simulink library "thermochemical"  (R2017b)
settings: Solver=VariableStepAuto  StartTime=0.0  StopTime=10.0  RelTol=1e-3
values from neighbouring files (symbols this model uses):
  c = conversion_factors()    [blk_clausius_clapeyron.m]    (also in blk_clausius_clapeyron_no_popup.m; blk_cold_room_closed_dry_air.m; blk_reactor_BaCl2_NH3_no_walls.m; blk_reactor_BaCl2_NH3_no_walls_state_space.m)
  cp = metal.cp    [blk_wall_simple.m]    (also in get_metal_properties.m = 390)
  fluid = get_param(blk,'fluid')    [blk_thermodynamic_properties_nonsaturated.m]    (also in blk_thermodynamic_properties_nonsaturated_interpreted.m; blk_thermodynamic_properties_saturated.m; blk_thermodynamic_properties_saturated_interpreted.m; blk_thermodynamic_properties_saturated_mix.m)
  gas = get_material_properties(x.gasName)    [blk_reactor_BaCl2_NH3_cylindrical_no_walls_fun1.m]
  h = get_param(gcb,'ObjectParameters')    [get_param_eval.m]
  rho = metal.rho    [blk_wall_simple.m]    (also in get_metal_properties.m = 8940)
  s = solve(eq,dx,'ReturnConditions',true)    [LMTD_inv.m]    (also in blk_wall_simple.m = get_param_eval(blk,'s'))
  u_gas_at_T_ref = -R * T_ref    [blk_reactor_BaCl2_NH3_no_walls.m]    (also in blk_reactor_BaCl2_NH3_no_walls_state_space.m)
undefined symbols (not defined in the file or in its folder): b_motor, BaCl2, beta, CoolProp, cP_binder, cP_gas, cP_s0, cv, dh_r_0, ENG, heat_exchanger_epsilonNTU_inv_simulink, heat_exchanger_epsilonNTU_simulink, J_motor, K_cin, kappa, Km_motor, La_motor, lookup2D_BreakPoint2, M_binder, N_binder, N_gas_free_volume_init, N_salt, NH3, nh3_v3, nu, P, phase, PID_D_motor, PID_I_motor, PID_P_motor, Ra_motor, Reactor_phase, T, T1, T2, T_init, Tr_init, Tr_ref, U_binder_at_Tr_ref, U_salt_at_X0_Tr_ref, Ur_init, V_void, Valve_regime, Vmax_motor, w_init_motor, X_init
libraries: thermochemical x247, simulink x54, dspsigops x3
(part 11 of 12)

== system thermochemical/Reactors/Reactor, BaCl2//NH3, state-space form, [Tr, Ng, X] as state variables, no algebraic loops, ideal gas in void volume, ideal gas in salt/Reactor, BaCl2//NH3, no walls, state-space form, [Tr, Ng, X] as state variables, no algebraic loops, ideal gas in void volume/Reactor, no walls, state space form/Reactor state-space functions/f3/f3 ==
  In6 : Inport
  In1 : Inport  Port=2
  In2 : Inport  Port=3
  Gain4 : Gain  Gain=nu*N_salt
  Gain7 : Gain  Gain=1/V_void
  Ideal gas equation of state : thermochemical/Thermodynamic fluid properties/Ideal gas equation of state  sel=P(T,rho)  R=8.3145  Pa_to_bar=1e-5  bar_to_Pa=1e5
      settings: SourceProductName=@ Thermochemical
  "Reaction kinetic, differential equation" : Subsystem
  Sum2 : Sum  Inputs=|+-
  Out2 : Outport
  wires:
  "Reaction kinetic, differential equation"/1(Out2) -> Out2/1  "dX/dt (1/sec)"
  Ideal gas equation of state/1 -> "Reaction kinetic, differential equation"/2(In2)
  Sum2/1 -> Gain7/1  "Ngas,void"
  Gain7/1 -> Ideal gas equation of state/2
  Gain4/1 -> Sum2/2
  In6/1 -> "Reaction kinetic, differential equation"/1(In1), Ideal gas equation of state/1  "T (K)"
  In1/1 -> Sum2/1  "Ngas,total (mol)"
  In2/1 -> Gain4/1, "Reaction kinetic, differential equation"/3(In3)  "X (0..1)"

== system thermochemical/Reactors/Reactor, BaCl2//NH3, state-space form, [Tr, Ng, X] as state variables, no algebraic loops, real gas in void volume, ideal gas in salt/Reactor, BaCl2//NH3, no walls, state-space form, [Tr, Ng, X] as state variables, no algebraic loops, real gas in void volume, ideal gas in salt/Reactor, no walls, state space form/Reactor state-space functions/f1/denominator ==
  In6 : Inport
  In3 : Inport  Port=2
  In4 : Inport  Port=3
  Gain4 : Gain  Gain=nu*N_salt
  Gain7 : Gain  Gain=1/V_void
  K1 : Constant  Value=N_salt*cP_s0 + N_binder*M_binder*cP_binder  VectorParams1D=off
  K2 : Constant  Value=cP_gas  VectorParams1D=off
  Product1 : Product
  Product4 : Product
  Sum : Sum  Inputs=3
  Sum5 : Sum  Inputs=|+-
  Thermodynamic property (non-saturated)1 : thermochemical/Thermodynamic fluid properties/Thermodynamic  property (non-saturated)  sel=cv(T,rho)  fluid=fluid  reciprocVar=-1  lookup2D_BreakPoint1=fluid.no_sat.T_rho_indep.var_indep.T  lookup2D_BreakPoint2=fluid.no_sat.T_rho_indep.var_indep.rho_molar  lookup2D_Data=fluid.no_sat.T_rho_indep.var_dep.Cv_molar
      settings: SourceProductName=@ Thermochemical
  Thermodynamic property (non-saturated)2 : thermochemical/Thermodynamic fluid properties/Thermodynamic  property (non-saturated)  sel=cp(T,rho)  fluid=fluid  reciprocVar=-1  lookup2D_BreakPoint1=fluid.no_sat.T_rho_indep.var_indep.T  lookup2D_BreakPoint2=fluid.no_sat.T_rho_indep.var_indep.rho_molar  lookup2D_Data=fluid.no_sat.T_rho_indep.var_dep.Cp_molar
      settings: SourceProductName=@ Thermochemical
  Out2 : Outport
  wires:
  K1/1 -> Sum/1  "(J/K)"
  Sum/1 -> Out2/1  "denominator (J/K)"
  Sum5/1 -> Gain7/1, Product4/2  "Ngas,void"
  In4/1 -> Gain4/1  "X (0..1)"
  In3/1 -> Sum5/1  "Ngas,total (mol)"
  Gain7/1 -> Thermodynamic property (non-saturated)2/2, Thermodynamic property (non-saturated)1/2  "rho (mol/m3)"
  In6/1 -> Thermodynamic property (non-saturated)2/1, Thermodynamic property (non-saturated)1/1  "T (K)"
  Thermodynamic property (non-saturated)1/1 -> Product4/1
  Product4/1 -> Sum/2  "(J/K)"
  Gain4/1 -> Product1/1, Sum5/2  "(mol gas/mol salt * mol salt = mol gas)"
  Thermodynamic property (non-saturated)2/1 -> ?
  Product1/1 -> Sum/3  "(J/K)"
  K2/1 -> Product1/2

== system thermochemical/Reactors/Reactor, BaCl2//NH3, state-space form, [Tr, Ng, X] as state variables, no algebraic loops, real gas in void volume, ideal gas in salt/Reactor, BaCl2//NH3, no walls, state-space form, [Tr, Ng, X] as state variables, no algebraic loops, real gas in void volume, ideal gas in salt/Reactor, no walls, state space form/Reactor state-space functions/f1/f1 ==
  In6 : Inport
  In1 : Inport  Port=2
  In2 : Inport  Port=3
  Gain4 : Gain  Gain=nu*N_salt
  Gain7 : Gain  Gain=1/V_void
  Sum2 : Sum  Inputs=|+-
  Thermodynamic property (non-saturated)1 : thermochemical/Thermodynamic fluid properties/Thermodynamic  property (non-saturated)  sel=h(T,rho)  fluid=fluid  reciprocVar=-1  lookup2D_BreakPoint1=fluid.no_sat.T_rho_indep.var_indep.T  lookup2D_BreakPoint2=fluid.no_sat.T_rho_indep.var_indep.rho_molar  lookup2D_Data=fluid.no_sat.T_rho_indep.var_dep.h_molar
      settings: SourceProductName=@ Thermochemical
  Out2 : Outport
  wires:
  Thermodynamic property (non-saturated)1/1 -> Out2/1  "h gas (J/mol)"
  Sum2/1 -> Gain7/1  "Ngas,void"
  Gain7/1 -> Thermodynamic property (non-saturated)1/2
  Gain4/1 -> Sum2/2
  In6/1 -> Thermodynamic property (non-saturated)1/1  "T (K)"
  In1/1 -> Sum2/1  "Ngas,total (mol)"
  In2/1 -> Gain4/1  "X (0..1)"

== system thermochemical/Reactors/Reactor, BaCl2//NH3, state-space form, [Tr, Ng, X] as state variables, no algebraic loops, real gas in void volume, ideal gas in salt/Reactor, BaCl2//NH3, no walls, state-space form, [Tr, Ng, X] as state variables, no algebraic loops, real gas in void volume, ideal gas in salt/Reactor, no walls, state space form/Reactor state-space functions/f1/f2 ==
  In6 : Inport
  In1 : Inport  Port=2
  In2 : Inport  Port=3
  Gain4 : Gain  Gain=nu*N_salt
  Gain7 : Gain  Gain=1/V_void
  Math Function : Math  Operator=reciprocal  SaturateOnIntegerOverflow=on
  Pressure conversion : thermochemical/Conversions/Pressure conversion  sel=bar --> Pa
      settings: SourceProductName=@ Thermochemical
  Product1 : Product
  Product4 : Product  Inputs=**/
  Sum5 : Sum  Inputs=|+-
  Sum6 : Sum  Inputs=|+-
  Sum7 : Sum  Inputs=|+-
  Thermodynamic property (non-saturated) : thermochemical/Thermodynamic fluid properties/Thermodynamic  property (non-saturated)  sel=u(T,rho)  fluid=fluid  reciprocVar=-1  lookup2D_BreakPoint1=fluid.no_sat.T_rho_indep.var_indep.T  lookup2D_BreakPoint2=fluid.no_sat.T_rho_indep.var_indep.rho_molar  lookup2D_Data=fluid.no_sat.T_rho_indep.var_dep.u_molar
      settings: SourceProductName=@ Thermochemical
  Thermodynamic property (non-saturated)1 : thermochemical/Thermodynamic fluid properties/Thermodynamic  property (non-saturated)  sel=beta(T,rho)  fluid=fluid  reciprocVar=-1  lookup2D_BreakPoint1=fluid.no_sat.T_rho_indep.var_indep.T  lookup2D_BreakPoint2=fluid.no_sat.T_rho_indep.var_indep.rho_molar  lookup2D_Data=fluid.no_sat.T_rho_indep.var_dep.beta
      settings: SourceProductName=@ Thermochemical
  Thermodynamic property (non-saturated)2 : thermochemical/Thermodynamic fluid properties/Thermodynamic  property (non-saturated)  sel=kappa(T,rho)  fluid=fluid  reciprocVar=-1  lookup2D_BreakPoint1=fluid.no_sat.T_rho_indep.var_indep.T  lookup2D_BreakPoint2=fluid.no_sat.T_rho_indep.var_indep.rho_molar  lookup2D_Data=fluid.no_sat.T_rho_indep.var_dep.kappa
      settings: SourceProductName=@ Thermochemical
  Thermodynamic property (non-saturated)3 : thermochemical/Thermodynamic fluid properties/Thermodynamic  property (non-saturated)  sel=P(T,rho)  fluid=fluid  reciprocVar=-1  lookup2D_BreakPoint1=fluid.no_sat.T_rho_indep.var_indep.T  lookup2D_BreakPoint2=fluid.no_sat.T_rho_indep.var_indep.rho_molar  lookup2D_Data=fluid.no_sat.T_rho_indep.var_dep.P
      settings: SourceProductName=@ Thermochemical
  Out2 : Outport
  wires:
  Pressure conversion/1 -> Sum7/2
  In6/1 -> Product4/1, Thermodynamic property (non-saturated)3/1, Thermodynamic property (non-saturated)2/1, Thermodynamic property (non-saturated)1/1, Thermodynamic property (non-saturated)/1  "T (K)"
  In1/1 -> Sum5/1  "Ngas,total (mol)"
  Gain4/1 -> Sum5/2
  In2/1 -> Gain4/1  "X (0..1)"
  Sum5/1 -> Gain7/1  "Ngas,void"
  Gain7/1 -> Math Function/1, Thermodynamic property (non-saturated)2/2, Thermodynamic property (non-saturated)3/2, Thermodynamic property (non-saturated)1/2, Thermodynamic property (non-saturated)/2  "rho (mol/m3)"
  Thermodynamic property (non-saturated)/1 -> Sum6/1  "u gas (J/mol)"
  Thermodynamic property (non-saturated)1/1 -> Product4/2
  Thermodynamic property (non-saturated)2/1 -> Product4/3
  Product4/1 -> Sum7/1
  Thermodynamic property (non-saturated)3/1 -> Pressure conversion/1
  Math Function/1 -> Product1/1
  Sum7/1 -> Product1/2
  Product1/1 -> Sum6/2  "(J/mol)"
  Sum6/1 -> Out2/1  "u - 1/rho*(T*beta/kappa-P) (J/mol)"

== system thermochemical/Reactors/Reactor, BaCl2//NH3, state-space form, [Tr, Ng, X] as state variables, no algebraic loops, real gas in void volume, ideal gas in salt/Reactor, BaCl2//NH3, no walls, state-space form, [Tr, Ng, X] as state variables, no algebraic loops, real gas in void volume, ideal gas in salt/Reactor, no walls, state space form/Reactor state-space functions/f1/f3 ==
  In6 : Inport
  In1 : Inport  Port=2
  In2 : Inport  Port=3
  Gain4 : Gain  Gain=nu*N_salt
  Gain7 : Gain  Gain=1/V_void
  "Reaction kinetic, differential equation" : Subsystem
  Sum2 : Sum  Inputs=|+-
  Thermodynamic property (non-saturated)1 : thermochemical/Thermodynamic fluid properties/Thermodynamic  property (non-saturated)  sel=P(T,rho)  fluid=fluid  reciprocVar=-1  lookup2D_BreakPoint1=fluid.no_sat.T_rho_indep.var_indep.T  lookup2D_BreakPoint2=fluid.no_sat.T_rho_indep.var_indep.rho_molar  lookup2D_Data=fluid.no_sat.T_rho_indep.var_dep.P
      settings: SourceProductName=@ Thermochemical
  Out2 : Outport
  wires:
  In2/1 -> "Reaction kinetic, differential equation"/3(In3), Gain4/1  "X (0..1)"
  In1/1 -> Sum2/1  "Ngas,total (mol)"
  In6/1 -> "Reaction kinetic, differential equation"/1(In1), Thermodynamic property (non-saturated)1/1  "T (K)"
  Gain4/1 -> Sum2/2
  Gain7/1 -> Thermodynamic property (non-saturated)1/2
  Sum2/1 -> Gain7/1  "Ngas,void"
  Thermodynamic property (non-saturated)1/1 -> "Reaction kinetic, differential equation"/2(In2)
  "Reaction kinetic, differential equation"/1(Out2) -> Out2/1  "dX/dt (1/sec)"

== system thermochemical/Reactors/Reactor, BaCl2//NH3, state-space form, [Tr, Ng, X] as state variables, no algebraic loops, real gas in void volume, real gas in salt/Reactor, BaCl2//NH3, no walls, state-space form, [Tr, Ng, X] as state variables, no algebraic loops, real gas in void volume, real gas in salt/Reactor, no walls, state space form/Reactor state-space functions/f1/denominator ==
  In6 : Inport
  In3 : Inport  Port=2
  In4 : Inport  Port=3
  Gain4 : Gain  Gain=nu*N_salt
  Gain7 : Gain  Gain=1/V_void
  K1 : Constant  Value=N_salt*cP_s0 + N_binder*M_binder*cP_binder  VectorParams1D=off
  Product1 : Product
  Product4 : Product
  Sum : Sum  Inputs=3
  Sum5 : Sum  Inputs=|+-
  Thermodynamic property (non-saturated)1 : thermochemical/Thermodynamic fluid properties/Thermodynamic  property (non-saturated)  sel=cv(T,rho)  fluid=fluid  reciprocVar=-1  lookup2D_BreakPoint1=fluid.no_sat.T_rho_indep.var_indep.T  lookup2D_BreakPoint2=fluid.no_sat.T_rho_indep.var_indep.rho_molar  lookup2D_Data=fluid.no_sat.T_rho_indep.var_dep.Cv_molar
      settings: SourceProductName=@ Thermochemical
  Thermodynamic property (non-saturated)2 : thermochemical/Thermodynamic fluid properties/Thermodynamic  property (non-saturated)  sel=cp(T,rho)  fluid=fluid  reciprocVar=-1  lookup2D_BreakPoint1=fluid.no_sat.T_rho_indep.var_indep.T  lookup2D_BreakPoint2=fluid.no_sat.T_rho_indep.var_indep.rho_molar  lookup2D_Data=fluid.no_sat.T_rho_indep.var_dep.Cp_molar
      settings: SourceProductName=@ Thermochemical
  Out2 : Outport
  wires:
  Product1/1 -> Sum/3  "(J/K)"
  Thermodynamic property (non-saturated)2/1 -> Product1/2
  Gain4/1 -> Sum5/2, Product1/1  "(mol gas/mol salt * mol salt = mol gas)"
  Product4/1 -> Sum/2  "(J/K)"
  Thermodynamic property (non-saturated)1/1 -> Product4/1
  In6/1 -> Thermodynamic property (non-saturated)1/1, Thermodynamic property (non-saturated)2/1  "T (K)"
  Gain7/1 -> Thermodynamic property (non-saturated)1/2, Thermodynamic property (non-saturated)2/2  "rho (mol/m3)"
  In3/1 -> Sum5/1  "Ngas,total (mol)"
  In4/1 -> Gain4/1  "X (0..1)"
  Sum5/1 -> Product4/2, Gain7/1  "Ngas,void"
  Sum/1 -> Out2/1  "denominator (J/K)"
  K1/1 -> Sum/1  "(J/K)"

== system thermochemical/Reactors/Reactor, BaCl2//NH3, state-space form, [Tr, Ng, X] as state variables, no algebraic loops, real gas in void volume, real gas in salt/Reactor, BaCl2//NH3, no walls, state-space form, [Tr, Ng, X] as state variables, no algebraic loops, real gas in void volume, real gas in salt/Reactor, no walls, state space form/Reactor state-space functions/f1/f1 ==
  In6 : Inport
  In1 : Inport  Port=2
  In2 : Inport  Port=3
  Gain4 : Gain  Gain=nu*N_salt
  Gain7 : Gain  Gain=1/V_void
  Sum2 : Sum  Inputs=|+-
  Thermodynamic property (non-saturated)1 : thermochemical/Thermodynamic fluid properties/Thermodynamic  property (non-saturated)  sel=h(T,rho)  fluid=fluid  reciprocVar=-1  lookup2D_BreakPoint1=fluid.no_sat.T_rho_indep.var_indep.T  lookup2D_BreakPoint2=fluid.no_sat.T_rho_indep.var_indep.rho_molar  lookup2D_Data=fluid.no_sat.T_rho_indep.var_dep.h_molar
      settings: SourceProductName=@ Thermochemical
  Out2 : Outport
  wires:
  In2/1 -> Gain4/1  "X (0..1)"
  In1/1 -> Sum2/1  "Ngas,total (mol)"
  In6/1 -> Thermodynamic property (non-saturated)1/1  "T (K)"
  Gain4/1 -> Sum2/2
  Gain7/1 -> Thermodynamic property (non-saturated)1/2
  Sum2/1 -> Gain7/1  "Ngas,void"
  Thermodynamic property (non-saturated)1/1 -> Out2/1  "h gas (J/mol)"

== system thermochemical/Reactors/Reactor, BaCl2//NH3, state-space form, [Tr, Ng, X] as state variables, no algebraic loops, real gas in void volume, real gas in salt/Reactor, BaCl2//NH3, no walls, state-space form, [Tr, Ng, X] as state variables, no algebraic loops, real gas in void volume, real gas in salt/Reactor, no walls, state space form/Reactor state-space functions/f1/f2 ==
  In6 : Inport
  In1 : Inport  Port=2
  In2 : Inport  Port=3
  Gain4 : Gain  Gain=nu*N_salt
  Gain7 : Gain  Gain=1/V_void
  Math Function : Math  Operator=reciprocal  SaturateOnIntegerOverflow=on
  Pressure conversion : thermochemical/Conversions/Pressure conversion  sel=bar --> Pa
      settings: SourceProductName=@ Thermochemical
  Product1 : Product
  Product4 : Product  Inputs=**/
  Sum5 : Sum  Inputs=|+-
  Sum6 : Sum  Inputs=|+-
  Sum7 : Sum  Inputs=|+-
  Thermodynamic property (non-saturated) : thermochemical/Thermodynamic fluid properties/Thermodynamic  property (non-saturated)  sel=u(T,rho)  fluid=fluid  reciprocVar=-1  lookup2D_BreakPoint1=fluid.no_sat.T_rho_indep.var_indep.T  lookup2D_BreakPoint2=fluid.no_sat.T_rho_indep.var_indep.rho_molar  lookup2D_Data=fluid.no_sat.T_rho_indep.var_dep.u_molar
      settings: SourceProductName=@ Thermochemical
  Thermodynamic property (non-saturated)1 : thermochemical/Thermodynamic fluid properties/Thermodynamic  property (non-saturated)  sel=beta(T,rho)  fluid=fluid  reciprocVar=-1  lookup2D_BreakPoint1=fluid.no_sat.T_rho_indep.var_indep.T  lookup2D_BreakPoint2=fluid.no_sat.T_rho_indep.var_indep.rho_molar  lookup2D_Data=fluid.no_sat.T_rho_indep.var_dep.beta
      settings: SourceProductName=@ Thermochemical
  Thermodynamic property (non-saturated)2 : thermochemical/Thermodynamic fluid properties/Thermodynamic  property (non-saturated)  sel=kappa(T,rho)  fluid=fluid  reciprocVar=-1  lookup2D_BreakPoint1=fluid.no_sat.T_rho_indep.var_indep.T  lookup2D_BreakPoint2=fluid.no_sat.T_rho_indep.var_indep.rho_molar  lookup2D_Data=fluid.no_sat.T_rho_indep.var_dep.kappa
      settings: SourceProductName=@ Thermochemical
  Thermodynamic property (non-saturated)3 : thermochemical/Thermodynamic fluid properties/Thermodynamic  property (non-saturated)  sel=P(T,rho)  fluid=fluid  reciprocVar=-1  lookup2D_BreakPoint1=fluid.no_sat.T_rho_indep.var_indep.T  lookup2D_BreakPoint2=fluid.no_sat.T_rho_indep.var_indep.rho_molar  lookup2D_Data=fluid.no_sat.T_rho_indep.var_dep.P
      settings: SourceProductName=@ Thermochemical
  Out2 : Outport
  wires:
  Sum6/1 -> Out2/1  "u - 1/rho*(T*beta/kappa-P) (J/mol)"
  Product1/1 -> Sum6/2  "(J/mol)"
  Sum7/1 -> Product1/2
  Math Function/1 -> Product1/1
  Thermodynamic property (non-saturated)3/1 -> Pressure conversion/1
  Product4/1 -> Sum7/1
  Thermodynamic property (non-saturated)2/1 -> Product4/3
  Thermodynamic property (non-saturated)1/1 -> Product4/2
  Thermodynamic property (non-saturated)/1 -> Sum6/1  "u gas (J/mol)"
  Gain7/1 -> Thermodynamic property (non-saturated)/2, Thermodynamic property (non-saturated)1/2, Thermodynamic property (non-saturated)3/2, Thermodynamic property (non-saturated)2/2, Math Function/1  "rho (mol/m3)"
  Sum5/1 -> Gain7/1  "Ngas,void"
  In2/1 -> Gain4/1  "X (0..1)"
  Gain4/1 -> Sum5/2
  In1/1 -> Sum5/1  "Ngas,total (mol)"
  In6/1 -> Thermodynamic property (non-saturated)/1, Thermodynamic property (non-saturated)1/1, Thermodynamic property (non-saturated)2/1, Thermodynamic property (non-saturated)3/1, Product4/1  "T (K)"
  Pressure conversion/1 -> Sum7/2

== system thermochemical/Reactors/Reactor, BaCl2//NH3, state-space form, [Tr, Ng, X] as state variables, no algebraic loops, real gas in void volume, real gas in salt/Reactor, BaCl2//NH3, no walls, state-space form, [Tr, Ng, X] as state variables, no algebraic loops, real gas in void volume, real gas in salt/Reactor, no walls, state space form/Reactor state-space functions/f1/f3 ==
  In6 : Inport
  In1 : Inport  Port=2
  In2 : Inport  Port=3
  Gain4 : Gain  Gain=nu*N_salt
  Gain7 : Gain  Gain=1/V_void
  "Reaction kinetic, differential equation" : Subsystem
  Sum2 : Sum  Inputs=|+-
  Thermodynamic property (non-saturated)1 : thermochemical/Thermodynamic fluid properties/Thermodynamic  property (non-saturated)  sel=P(T,rho)  fluid=fluid  reciprocVar=-1  lookup2D_BreakPoint1=fluid.no_sat.T_rho_indep.var_indep.T  lookup2D_BreakPoint2=fluid.no_sat.T_rho_indep.var_indep.rho_molar  lookup2D_Data=fluid.no_sat.T_rho_indep.var_dep.P
      settings: SourceProductName=@ Thermochemical
  Out2 : Outport
  wires:
  "Reaction kinetic, differential equation"/1(Out2) -> Out2/1  "dX/dt (1/sec)"
  Thermodynamic property (non-saturated)1/1 -> "Reaction kinetic, differential equation"/2(In2)
  Sum2/1 -> Gain7/1  "Ngas,void"
  Gain7/1 -> Thermodynamic property (non-saturated)1/2
  Gain4/1 -> Sum2/2
  In6/1 -> Thermodynamic property (non-saturated)1/1, "Reaction kinetic, differential equation"/1(In1)  "T (K)"
  In1/1 -> Sum2/1  "Ngas,total (mol)"
  In2/1 -> Gain4/1, "Reaction kinetic, differential equation"/3(In3)  "X (0..1)"

== system thermochemical/Reactors/Reactor, BaCl2//NH3, state-space form, [Tr, Ng, X] as state variables, no algebraic loops, real gas in void volume, real gas in salt/Reactor, BaCl2//NH3, no walls, state-space form, [Tr, Ng, X] as state variables, no algebraic loops, real gas in void volume, real gas in salt/Reactor, no walls, state space form/Reactor state-space functions/f1/f4 ==
  In6 : Inport
  Clausius-Clapeyron1 : thermochemical/Thermodynamic fluid properties/Clausius-Clapeyron  sel_1=P(T)  sel_2=BaCl2/NH3
      settings: SourceProductName=@ Thermochemical
  Enthalpy of reaction per mole of gas : Constant  Value=dh_r_0  VectorParams1D=off
  Sum : Sum  Inputs=-+
  Thermodynamic property (non-saturated)1 : thermochemical/Thermodynamic fluid properties/Thermodynamic  property (non-saturated)  sel=h(T,P)  fluid=fluid  reciprocVar=-1  lookup2D_BreakPoint1=fluid.no_sat.T_P_indep.var_indep.T  lookup2D_BreakPoint2=fluid.no_sat.T_P_indep.var_indep.P  lookup2D_Data=fluid.no_sat.T_P_indep.var_dep.h_molar
      settings: SourceProductName=@ Thermochemical
  Out2 : Outport
  wires:
  Enthalpy of reaction per mole of gas/1 -> Sum/1  "(J/mol of gas)"
  Sum/1 -> Out2/1  "(J/mol gas)"
  In6/1 -> Thermodynamic property (non-saturated)1/1, Clausius-Clapeyron1/1  "Tr (K)"
  Clausius-Clapeyron1/1 -> Thermodynamic property (non-saturated)1/2
  Thermodynamic property (non-saturated)1/1 -> Sum/2  "h gas[Tr,Peq(Tr)] (J/mol)"

== system thermochemical/Reactors/Reactor, BaCl2//NH3, state-space form, [Ur, Ng, X] as state variables, no algebraic loops, ideal gas in void volume, ideal gas in salt/Reactor, BaCl2//NH3, no walls, state-space form, [Ur, Ng, X] as state variables, no algebraic loops, ideal gas in void volume, ideal gas in salt/Reactor, no walls, state space form/Reactor state-space functions/f1/Reactor's internal energy differential equation ==
  In1 : Inport
  In2 : Inport  Port=2
  In5 : Inport  Port=3
  In3 : Inport  Port=4
  Product4 : Product
  Relay : Relay  OnSwitchValue=dn_dead_zone  OffSwitchValue=-dn_dead_zone  OffOutputValue=-1
  Sum19 : Sum  Inputs=++|
  Switch1 : Switch
  Out1 : Outport
  wires:
  In3/1 -> Relay/1, Product4/2  "dn_gas (mol/sec) > 0: gas in   < 0: gas out"
  In5/1 -> Switch1/3  "enthalpy out (J/mol)"
  In1/1 -> Sum19/1  "q out → in (W)"
  Sum19/1 -> Out1/1  "dUr/dt (J/sec)"
  In2/1 -> Switch1/1  "enthalpy in (J/mol)"
  Switch1/1 -> Product4/1  "h_gas(Tgas)"
  Product4/1 -> Sum19/2  "dn_gas * h_gas"
  Relay/1 -> Switch1/2

== system thermochemical/Reactors/Reactor, BaCl2//NH3, state-space form, [Ur, Ng, X] as state variables, no algebraic loops, ideal gas in void volume, ideal gas in salt/Reactor, BaCl2//NH3, no walls, state-space form, [Ur, Ng, X] as state variables, no algebraic loops, ideal gas in void volume, ideal gas in salt/Reactor, no walls, state space form/Reactor state-space functions/f1/Tr = inv(g[X(vector)]) ==
  In6 : Inport
  In3 : Inport  Port=2
  In4 : Inport  Port=3
  Constant : Constant  Value=N_salt*cP_s0 + N_binder*M_binder*cP_binder  VectorParams1D=off
  Constant1 : Constant  Value=U_salt_at_X0_T_ref  VectorParams1D=off
  Constant2 : Constant  Value=U_binder_at_T_ref  VectorParams1D=off
  Cp gas : Gain  Gain=cP_gas
  Cv gas : Gain  Gain=cP_gas - R
  Gain1 : Gain  Gain=R * T_ref - dh_r_0
  Gain2 : Gain  Gain=u_gas_at_T_ref
  Gain4 : Gain  Gain=nu*N_salt
  K5 : Constant  Value=T_ref  VectorParams1D=off
  Product2 : Product  Inputs=*/
  Sum : Sum  Inputs=3
  Sum1 : Sum  Inputs=++++
  Sum2 : Sum  Inputs=|++
  Sum3 : Sum  Inputs=|+-
  Sum4 : Sum  Inputs=|+-
  Out2 : Outport
  wires:
  In6/1 -> Sum3/1  "Ur (J)"
  Constant/1 -> Sum/1  "(J/K)"
  Sum2/1 -> Out2/1  "Tr (K)"
  In4/1 -> Gain4/1  "X (0..1)"
  In3/1 -> Gain2/1, Sum4/1  "Ngas,total (mol)"
  Cv gas/1 -> Sum/2  "(J/K)"
  Gain4/1 -> Gain1/1, Sum4/2, Cp gas/1  "(mol gas/mol salt * mol salt = mol gas)"
  Cp gas/1 -> Sum/3  "(J/K)"
  K5/1 -> Sum2/2
  Sum/1 -> Product2/2  "denominator (J/K)"
  Gain1/1 -> Sum1/4  "mol*(J/mol/K * K - J/mol)"
  Sum3/1 -> Product2/1  "numerator (J)"
  Product2/1 -> Sum2/1  "(K)"
  Sum4/1 -> Cv gas/1
  Sum1/1 -> Sum3/2  "(J)"
  Gain2/1 -> Sum1/1  "(J)"
  Constant1/1 -> Sum1/2  "(J)"
  Constant2/1 -> Sum1/3  "(J)"

== system thermochemical/Reactors/Reactor, BaCl2//NH3, state-space form, [Ur, Ng, X] as state variables, no algebraic loops, ideal gas in void volume, ideal gas in salt/Reactor, BaCl2//NH3, no walls, state-space form, [Ur, Ng, X] as state variables, no algebraic loops, ideal gas in void volume, ideal gas in salt/Reactor, no walls, state space form/Reactor state-space functions/f3/f3 ==
  In6 : Inport
  In1 : Inport  Port=2
  In2 : Inport  Port=3
  Gain4 : Gain  Gain=nu*N_salt
  Gain7 : Gain  Gain=1/V_void
  Ideal gas equation of state : thermochemical/Thermodynamic fluid properties/Ideal gas equation of state  sel=P(T,rho)  R=8.3145  Pa_to_bar=1e-5  bar_to_Pa=1e5
      settings: SourceProductName=@ Thermochemical
  "Reaction kinetic, differential equation" : Subsystem
  Sum2 : Sum  Inputs=|+-
  Out2 : Outport
  wires:
  In2/1 -> "Reaction kinetic, differential equation"/3(In3), Gain4/1  "X (0..1)"
  In1/1 -> Sum2/1  "Ngas,total (mol)"
  In6/1 -> Ideal gas equation of state/1, "Reaction kinetic, differential equation"/1(In1)  "T (K)"
  Gain4/1 -> Sum2/2
  Gain7/1 -> Ideal gas equation of state/2
  Sum2/1 -> Gain7/1  "Ngas,void"
  Ideal gas equation of state/1 -> "Reaction kinetic, differential equation"/2(In2)
  "Reaction kinetic, differential equation"/1(Out2) -> Out2/1  "dX/dt"

== system thermochemical/Reactors/Reactor, BaCl2//NH3, with algebraic loops, ideal gas in void volume, ideal gas in salt/Reactor, BaCl2//NH3, no walls, with algebraic loops, ideal gas in void volume, ideal gas in salt/Reactor (no walls)/Reactor's temperature and pressure/Reaction kinetic, differential equation/Reaction kinetic, differential equation ==
  note: Desorption
  note: Synthesis
  In1 : Inport
  In2 : Inport  Port=2
  In3 : Inport  Port=3
  3 : Constant
  Clausius-Clapeyron : thermochemical/Thermodynamic fluid properties/Clausius-Clapeyron  sel_1=P(T)  sel_2=BaCl2/NH3
      settings: SourceProductName=@ Thermochemical
  Divide1 : Product  Inputs=/*
  Gain15 : Gain  Gain=K_cin
  Product6 : Product
  Relay : Relay  OnSwitchValue=P_dead_zone  OffSwitchValue=-P_dead_zone  OffOutputValue=-1
  Sum16 : Sum  Inputs=+-
  Sum17 : Sum  Inputs=+-|
  Switch : Switch  Criteria=u2 > Threshold
  Out2 : Outport
  wires:
  Sum17/1 -> Switch/1  "1 - X"
  Divide1/1 -> Gain15/1
  Switch/1 -> Product6/2
  In2/1 -> Sum16/1, Divide1/1  "P (bar)"
  Product6/1 -> Out2/1  "dX/dt"
  3/1 -> Sum17/1
  Gain15/1 -> Product6/1
  Clausius-Clapeyron/1 -> Sum16/2  "P_equilb (bar)"
  Sum16/1 -> Relay/1, Divide1/2  "dP"
  In1/1 -> Clausius-Clapeyron/1  "T(K)"
  Relay/1 -> Switch/2
  In3/1 -> Sum17/2, Switch/3  "X (0..1)"

== system thermochemical/Reactors/Reactor, BaCl2//NH3, with algebraic loops, ideal gas in void volume, ideal gas in salt/Reactor, BaCl2//NH3, no walls, with algebraic loops, ideal gas in void volume, ideal gas in salt/Reactor (no walls)/Reactor's temperature and pressure/Reaction kinetic, differential equation/Reactor phase ==
  In1 : Inport
  3 : Constant  Value=P_dead_zone
  Abs : Abs
  Enumerated Constant : simulink/Sources/Enumerated Constant  OutDataTypeStr=Enum: Reactor_phase  Value=Reactor_phase.Synthesis  SampleTime=inf
      settings: SourceProductName=Simulink
  Enumerated Constant1 : simulink/Sources/Enumerated Constant  OutDataTypeStr=Enum: Reactor_phase  Value=Reactor_phase.Desorption  SampleTime=inf
      settings: SourceProductName=Simulink
  Enumerated Constant2 : simulink/Sources/Enumerated Constant  OutDataTypeStr=Enum: Reactor_phase  Value=Reactor_phase.No_reaction  SampleTime=inf
      settings: SourceProductName=Simulink
  Relay : Relay  OnSwitchValue=P_dead_zone  OffSwitchValue=-P_dead_zone  OffOutputValue=-1
  Sign : Signum
  Sum17 : Sum  Inputs=|+-
  Switch1 : Switch  Criteria=u2 > Threshold
  Switch2 : Switch  Criteria=u2 > Threshold
  Out1 : Outport
  wires:
  Switch2/1 -> Out1/1  "Reactor phase"
  Enumerated Constant/1 -> Switch1/1  "Synthesis"
  Enumerated Constant1/1 -> Switch1/3  "Decomposition (desporption)"
  Switch1/1 -> Switch2/1
  Enumerated Constant2/1 -> Switch2/3  "No reaction"
  In1/1 -> Relay/1, Abs/1  "dP"
  Relay/1 -> Switch1/2
  Sum17/1 -> Sign/1
  Abs/1 -> Sum17/1
  Sign/1 -> Switch2/2
  3/1 -> Sum17/2

== system thermochemical/Reactors/Reactor, BaCl2//NH3, with algebraic loops, ideal gas in void volume, ideal gas in salt/Reactor, BaCl2//NH3, no walls, with algebraic loops, ideal gas in void volume, ideal gas in salt/Reactor (no walls)/Reactor's temperature and pressure/Reactor's energy balance/Temperature equation ==
  note: The error must be ~ 0
      | (1e-9 is more that fine!)
  note: The "algebraic constraint"
      | block computes the reactor's
      | temperature by feeding back
      | its value to the "Reactor
      | energy balance" block until
      | the error between the input
      | and computed reactor's internal
      | energy (U_reactor) is zero. This
      | is done at every simulation step.
      |
      | This is a way to compute the inverse
      | of a function. In our case, we have
      | the "Reactor energy balance" block,
      | which computes the Energy as a function
      | of the Temperature. But we have the
      | Energ and we want to compute the
      | Temperature.
  In1 : Inport
  In2 : Inport  Port=2
  In3 : Inport  Port=3
  Algebraic Constraint : AlgebraicConstraint  InitialGuess=Tr_init
  Check Dynamic Range : simulink/Model Verification/Check  Dynamic Range  Description=min < u < max  enabled=on  stopWhenAssertionFail=on  export=off  icon=graphic
      settings: SourceProductName=Simulink  SourceProductBaseCode=SL
  Display : Display
  Reactor's internal energy equation : thermochemical/Reactors/Reactor's internal energy equation  Tr_ref=T_ref  N_salt=N_salt  cP_s0=cP_s0  U_salt_at_X0_Tr_ref=U_salt_at_X0_T_ref  N_binder=N_binder  M_binder=M_binder  cP_binder=cP_binder  U_binder_at_Tr_ref=U_binder_at_T_ref  V_void=V_void  gas_model_void_volume=Ideal gas model  gas_model_salt=Ideal gas model  is_ideal_gas_in_void_volume=1  is_ideal_gas_in_salt=1  fluid=fluid  cP_gas=cP_gas  u_gas_at_Tr_ref=u_gas_at_T_ref  nu=nu  dh_r=dh_r_0  R=8.314472
      settings: SourceProductName=@ Thermochemical
  Scope14 : Scope
  Sum20 : Sum  Inputs=+-|
  dn_gas2 : Constant  Value=fluid.constants.Tmax
  dn_gas4 : Constant  Value=fluid.constants.Tmin
  Out1 : Outport
  wires:
  In3/1 -> Reactor's internal energy equation/2  "N_gas_free_volume (mol)"
  Reactor's internal energy equation/1 -> Sum20/2
  In2/1 -> Reactor's internal energy equation/1  "X ([0..1])"
  dn_gas2/1 -> Check Dynamic Range/1
  Sum20/1 -> Algebraic Constraint/1, Scope14/1, Display/1  "error"
  dn_gas4/1 -> Check Dynamic Range/2
  In1/1 -> Sum20/1  "U_reactor (J)"
  Algebraic Constraint/1 -> Reactor's internal energy equation/3, Out1/1, Check Dynamic Range/3  "T_reactor (K)"

== system thermochemical/Reactors/Reactor, BaCl2//NH3, with algebraic loops, ideal gas in void volume, ideal gas in salt/Reactor, BaCl2//NH3, no walls, with algebraic loops, ideal gas in void volume, ideal gas in salt/Reactor (no walls)/Reactor's temperature and pressure/Reactor's energy balance/Void volume pressure equation (real model) ==
  note: The ideal gas model is presented here
      | just for the sake of comparison,
      | but it is not used outside this block.
  In2 : Inport
  In1 : Inport  Port=2
  Gain1 : Gain  Gain=1/V_void
  Ideal gas equation of state : thermochemical/Thermodynamic fluid properties/Ideal gas equation of state  sel=P(T,rho)  R=8.3145  Pa_to_bar=1e-5  bar_to_Pa=1e5
      settings: SourceProductName=@ Thermochemical
  Mux1 : Mux  Inputs=2
  P(T,rho) : thermochemical/Thermodynamic fluid properties/Thermodynamic  property (non-saturated)  sel=P(T,rho)  fluid=fluid  reciprocVar=-1  lookup2D_BreakPoint1=fluid.no_sat.T_rho_indep.var_indep.T  lookup2D_BreakPoint2=fluid.no_sat.T_rho_indep.var_indep.rho_molar  lookup2D_Data=fluid.no_sat.T_rho_indep.var_dep.P
      settings: SourceProductName=@ Thermochemical
  Terminator : Terminator
  Out1 : Outport
  wires:
  Mux1/1 -> Terminator/1  "Comparison"
  Ideal gas equation of state/1 -> Out1/1, Mux1/2  "P_reactor ideal (bar)"
  P(T,rho)/1 -> Mux1/1  "P_reactor (bar)"
  Gain1/1 -> Ideal gas equation of state/2, P(T,rho)/2  "rho_molar (mol/m3)"
  In2/1 -> Ideal gas equation of state/1, P(T,rho)/1  "T (K)"
  In1/1 -> Gain1/1  "N (mol)"

== system thermochemical/Reactors/Reactor, BaCl2//NH3, with algebraic loops, real gas in void volume, ideal gas in salt/Reactor, BaCl2//NH3, no walls, with algebraic loops, real gas in void volume, ideal gas in salt/Reactor (no walls)/Reactor's temperature and pressure/Reaction kinetic, differential equation/Reaction kinetic, differential equation ==
  note: Synthesis
  note: Desorption
  In1 : Inport
  In2 : Inport  Port=2
  In3 : Inport  Port=3
  3 : Constant
  Clausius-Clapeyron : thermochemical/Thermodynamic fluid properties/Clausius-Clapeyron  sel_1=P(T)  sel_2=BaCl2/NH3
      settings: SourceProductName=@ Thermochemical
  Divide1 : Product  Inputs=/*
  Gain15 : Gain  Gain=K_cin
  Product6 : Product
  Relay : Relay  OnSwitchValue=P_dead_zone  OffSwitchValue=-P_dead_zone  OffOutputValue=-1
  Sum16 : Sum  Inputs=+-
  Sum17 : Sum  Inputs=+-|
  Switch : Switch  Criteria=u2 > Threshold
  Out2 : Outport
  wires:
  In3/1 -> Switch/3, Sum17/2  "X (0..1)"
  Relay/1 -> Switch/2
  In1/1 -> Clausius-Clapeyron/1  "T(K)"
  Sum16/1 -> Divide1/2, Relay/1  "dP"
  Clausius-Clapeyron/1 -> Sum16/2  "P_equilb (bar)"
  Gain15/1 -> Product6/1
  3/1 -> Sum17/1
  Product6/1 -> Out2/1  "dX/dt"
  In2/1 -> Divide1/1, Sum16/1  "P (bar)"
  Switch/1 -> Product6/2
  Divide1/1 -> Gain15/1
  Sum17/1 -> Switch/1  "1 - X"

== system thermochemical/Reactors/Reactor, BaCl2//NH3, with algebraic loops, real gas in void volume, ideal gas in salt/Reactor, BaCl2//NH3, no walls, with algebraic loops, real gas in void volume, ideal gas in salt/Reactor (no walls)/Reactor's temperature and pressure/Reaction kinetic, differential equation/Reactor phase ==
  In1 : Inport
  3 : Constant  Value=P_dead_zone
  Abs : Abs
  Enumerated Constant : simulink/Sources/Enumerated Constant  OutDataTypeStr=Enum: Reactor_phase  Value=Reactor_phase.Synthesis  SampleTime=inf
      settings: SourceProductName=Simulink
  Enumerated Constant1 : simulink/Sources/Enumerated Constant  OutDataTypeStr=Enum: Reactor_phase  Value=Reactor_phase.Desorption  SampleTime=inf
      settings: SourceProductName=Simulink
  Enumerated Constant2 : simulink/Sources/Enumerated Constant  OutDataTypeStr=Enum: Reactor_phase  Value=Reactor_phase.No_reaction  SampleTime=inf
      settings: SourceProductName=Simulink
  Relay : Relay  OnSwitchValue=P_dead_zone  OffSwitchValue=-P_dead_zone  OffOutputValue=-1
  Sign : Signum
  Sum17 : Sum  Inputs=|+-
  Switch1 : Switch  Criteria=u2 > Threshold
  Switch2 : Switch  Criteria=u2 > Threshold
  Out1 : Outport
  wires:
  3/1 -> Sum17/2
  Sign/1 -> Switch2/2
  Abs/1 -> Sum17/1
  Sum17/1 -> Sign/1
  Relay/1 -> Switch1/2
  In1/1 -> Abs/1, Relay/1  "dP"
  Enumerated Constant2/1 -> Switch2/3  "No reaction"
  Switch1/1 -> Switch2/1
  Enumerated Constant1/1 -> Switch1/3  "Decomposition (desporption)"
  Enumerated Constant/1 -> Switch1/1  "Synthesis"
  Switch2/1 -> Out1/1  "Reactor phase"

== system thermochemical/Reactors/Reactor, BaCl2//NH3, with algebraic loops, real gas in void volume, ideal gas in salt/Reactor, BaCl2//NH3, no walls, with algebraic loops, real gas in void volume, ideal gas in salt/Reactor (no walls)/Reactor's temperature and pressure/Reactor's energy balance/Temperature equation ==
  note: The "algebraic constraint"
      | block computes the reactor's
      | temperature by feeding back
      | its value to the "Reactor
      | energy balance" block until
      | the error between the input
      | and computed reactor's internal
      | energy (U_reactor) is zero. This
      | is done at every simulation step.
      |
      | This is a way to compute the inverse
      | of a function. In our case, we have
      | the "Reactor energy balance" block,
      | which computes the Energy as a function
      | of the Temperature. But we have the
      | Energ and we want to compute the
      | Temperature.
  note: The error must be ~ 0
      | (1e-9 is more that fine!)
  In1 : Inport
  In2 : Inport  Port=2
  In3 : Inport  Port=3
  Algebraic Constraint : AlgebraicConstraint  InitialGuess=Tr_init
  Check Dynamic Range : simulink/Model Verification/Check  Dynamic Range  Description=min < u < max  enabled=on  stopWhenAssertionFail=on  export=off  icon=graphic
      settings: SourceProductName=Simulink  SourceProductBaseCode=SL
  Display : Display
  Reactor's internal energy equation : thermochemical/Reactors/Reactor's internal energy equation  Tr_ref=T_ref  N_salt=N_salt  cP_s0=cP_s0  U_salt_at_X0_Tr_ref=U_salt_at_X0_T_ref  N_binder=N_binder  M_binder=M_binder  cP_binder=cP_binder  U_binder_at_Tr_ref=U_binder_at_T_ref  V_void=V_void  gas_model_void_volume=Real gas model  gas_model_salt=Ideal gas model  is_ideal_gas_in_void_volume=-1  is_ideal_gas_in_salt=1  fluid=fluid  cP_gas=cP_gas  u_gas_at_Tr_ref=u_gas_at_T_ref  nu=nu  dh_r=dh_r_0  R=8.314472
      settings: SourceProductName=@ Thermochemical
  Scope14 : Scope
  Sum20 : Sum  Inputs=+-|
  dn_gas2 : Constant  Value=fluid.constants.Tmax
  dn_gas4 : Constant  Value=fluid.constants.Tmin
  Out1 : Outport
  wires:
  Algebraic Constraint/1 -> Check Dynamic Range/3, Out1/1, Reactor's internal energy equation/3  "T_reactor (K)"
  In1/1 -> Sum20/1  "U_reactor (J)"
  dn_gas4/1 -> Check Dynamic Range/2
  Sum20/1 -> Display/1, Scope14/1, Algebraic Constraint/1  "error"
  dn_gas2/1 -> Check Dynamic Range/1
  In2/1 -> Reactor's internal energy equation/1  "X ([0..1])"
  Reactor's internal energy equation/1 -> Sum20/2
  In3/1 -> Reactor's internal energy equation/2  "N_gas_free_volume (mol)"

== system thermochemical/Reactors/Reactor, BaCl2//NH3, with algebraic loops, real gas in void volume, ideal gas in salt/Reactor, BaCl2//NH3, no walls, with algebraic loops, real gas in void volume, ideal gas in salt/Reactor (no walls)/Reactor's temperature and pressure/Reactor's energy balance/Void volume pressure equation (real model) ==
  note: The ideal gas model is presented here
      | just for the sake of comparison,
      | but it is not used outside this block.
  In2 : Inport
  In1 : Inport  Port=2
  Gain1 : Gain  Gain=1/V_void
  Ideal gas equation of state : thermochemical/Thermodynamic fluid properties/Ideal gas equation of state  sel=P(T,rho)  R=8.3145  Pa_to_bar=1e-5  bar_to_Pa=1e5
      settings: SourceProductName=@ Thermochemical
  Mux1 : Mux  Inputs=2
  P(T,rho) : thermochemical/Thermodynamic fluid properties/Thermodynamic  property (non-saturated)  sel=P(T,rho)  fluid=fluid  reciprocVar=-1  lookup2D_BreakPoint1=fluid.no_sat.T_rho_indep.var_indep.T  lookup2D_BreakPoint2=fluid.no_sat.T_rho_indep.var_indep.rho_molar  lookup2D_Data=fluid.no_sat.T_rho_indep.var_dep.P
      settings: SourceProductName=@ Thermochemical
  Terminator : Terminator
  Out1 : Outport
  wires:
  In1/1 -> Gain1/1  "N (mol)"
  In2/1 -> P(T,rho)/1, Ideal gas equation of state/1  "T (K)"
  Gain1/1 -> P(T,rho)/2, Ideal gas equation of state/2  "rho_molar (mol/m3)"
  P(T,rho)/1 -> Out1/1, Mux1/1  "P_reactor (bar)"
  Ideal gas equation of state/1 -> Mux1/2  "P_reactor ideal (bar)"
  Mux1/1 -> Terminator/1  "Comparison"

== system thermochemical/Reactors/Reactor, BaCl2//NH3, with algebraic loops, real gas in void volume, real gas in salt/Reactor, BaCl2//NH3, no walls, with algebraic loops, real gas in void volume, real gas in salt/Reactor (no walls)/Reactor's temperature and pressure/Reaction kinetic, differential equation/Reaction kinetic, differential equation ==
  note: Desorption
  note: Synthesis
  In1 : Inport
  In2 : Inport  Port=2
  In3 : Inport  Port=3
  3 : Constant
  Clausius-Clapeyron : thermochemical/Thermodynamic fluid properties/Clausius-Clapeyron  sel_1=P(T)  sel_2=BaCl2/NH3
      settings: SourceProductName=@ Thermochemical
  Divide1 : Product  Inputs=/*
  Gain15 : Gain  Gain=K_cin
  Product6 : Product
  Relay : Relay  OnSwitchValue=P_dead_zone  OffSwitchValue=-P_dead_zone  OffOutputValue=-1
  Sum16 : Sum  Inputs=+-
  Sum17 : Sum  Inputs=+-|
  Switch : Switch  Criteria=u2 > Threshold
  Out2 : Outport
  wires:
  Sum17/1 -> Switch/1  "1 - X"
  Divide1/1 -> Gain15/1
  Switch/1 -> Product6/2
  In2/1 -> Sum16/1, Divide1/1  "P (bar)"
  Product6/1 -> Out2/1  "dX/dt"
  3/1 -> Sum17/1
  Gain15/1 -> Product6/1
  Clausius-Clapeyron/1 -> Sum16/2  "P_equilb (bar)"
  Sum16/1 -> Relay/1, Divide1/2  "dP"
  In1/1 -> Clausius-Clapeyron/1  "T(K)"
  Relay/1 -> Switch/2
  In3/1 -> Sum17/2, Switch/3  "X (0..1)"

== system thermochemical/Reactors/Reactor, BaCl2//NH3, with algebraic loops, real gas in void volume, real gas in salt/Reactor, BaCl2//NH3, no walls, with algebraic loops, real gas in void volume, real gas in salt/Reactor (no walls)/Reactor's temperature and pressure/Reaction kinetic, differential equation/Reactor phase ==
  In1 : Inport
  3 : Constant  Value=P_dead_zone
  Abs : Abs
  Enumerated Constant : simulink/Sources/Enumerated Constant  OutDataTypeStr=Enum: Reactor_phase  Value=Reactor_phase.Synthesis  SampleTime=inf
      settings: SourceProductName=Simulink
  Enumerated Constant1 : simulink/Sources/Enumerated Constant  OutDataTypeStr=Enum: Reactor_phase  Value=Reactor_phase.Desorption  SampleTime=inf
      settings: SourceProductName=Simulink
  Enumerated Constant2 : simulink/Sources/Enumerated Constant  OutDataTypeStr=Enum: Reactor_phase  Value=Reactor_phase.No_reaction  SampleTime=inf
      settings: SourceProductName=Simulink
  Relay : Relay  OnSwitchValue=P_dead_zone  OffSwitchValue=-P_dead_zone  OffOutputValue=-1
  Sign : Signum
  Sum17 : Sum  Inputs=|+-
  Switch1 : Switch  Criteria=u2 > Threshold
  Switch2 : Switch  Criteria=u2 > Threshold
  Out1 : Outport
  wires:
  Switch2/1 -> Out1/1  "Reactor phase"
  Enumerated Constant/1 -> Switch1/1  "Synthesis"
  Enumerated Constant1/1 -> Switch1/3  "Decomposition (desporption)"
  Switch1/1 -> Switch2/1
  Enumerated Constant2/1 -> Switch2/3  "No reaction"
  In1/1 -> Relay/1, Abs/1  "dP"
  Relay/1 -> Switch1/2
  Sum17/1 -> Sign/1
  Abs/1 -> Sum17/1
  Sign/1 -> Switch2/2
  3/1 -> Sum17/2

== system thermochemical/Reactors/Reactor, BaCl2//NH3, with algebraic loops, real gas in void volume, real gas in salt/Reactor, BaCl2//NH3, no walls, with algebraic loops, real gas in void volume, real gas in salt/Reactor (no walls)/Reactor's temperature and pressure/Reactor's energy balance/Temperature equation ==
  note: The error must be ~ 0
      | (1e-9 is more that fine!)
  note: The "algebraic constraint"
      | block computes the reactor's
      | temperature by feeding back
      | its value to the "Reactor
      | energy balance" block until
      | the error between the input
      | and computed reactor's internal
      | energy (U_reactor) is zero. This
      | is done at every simulation step.
      |
      | This is a way to compute the inverse
      | of a function. In our case, we have
      | the "Reactor energy balance" block,
      | which computes the Energy as a function
      | of the Temperature. But we have the
      | Energ and we want to compute the
      | Temperature.
  In1 : Inport
  In2 : Inport  Port=2
  In3 : Inport  Port=3
  Algebraic Constraint : AlgebraicConstraint  InitialGuess=Tr_init
  Check Dynamic Range : simulink/Model Verification/Check  Dynamic Range  Description=min < u < max  enabled=on  stopWhenAssertionFail=on  export=off  icon=graphic
      settings: SourceProductName=Simulink  SourceProductBaseCode=SL
  Display : Display
  Reactor's internal energy equation : thermochemical/Reactors/Reactor's internal energy equation  Tr_ref=T_ref  N_salt=N_salt  cP_s0=cP_s0  U_salt_at_X0_Tr_ref=U_salt_at_X0_T_ref  N_binder=N_binder  M_binder=M_binder  cP_binder=cP_binder  U_binder_at_Tr_ref=U_binder_at_T_ref  V_void=V_void  gas_model_void_volume=Real gas model  gas_model_salt=Real gas model  is_ideal_gas_in_void_volume=-1  is_ideal_gas_in_salt=-1  fluid=fluid  cP_gas=cP_gas  u_gas_at_Tr_ref=u_gas_at_T_ref  nu=nu  dh_r=dh_r_0  R=8.314472
      settings: SourceProductName=@ Thermochemical
  Scope14 : Scope
  Sum20 : Sum  Inputs=+-|
  dn_gas2 : Constant  Value=fluid.constants.Tmax
  dn_gas4 : Constant  Value=fluid.constants.Tmin
  Out1 : Outport
  wires:
  In3/1 -> Reactor's internal energy equation/2  "N_gas_free_volume (mol)"
  Reactor's internal energy equation/1 -> Sum20/2
  In2/1 -> Reactor's internal energy equation/1  "X ([0..1])"
  dn_gas2/1 -> Check Dynamic Range/1
  Sum20/1 -> Algebraic Constraint/1, Scope14/1, Display/1  "error"
  dn_gas4/1 -> Check Dynamic Range/2
  In1/1 -> Sum20/1  "U_reactor (J)"
  Algebraic Constraint/1 -> Reactor's internal energy equation/3, Out1/1, Check Dynamic Range/3  "T_reactor (K)"

== system thermochemical/Reactors/Reactor, BaCl2//NH3, with algebraic loops, real gas in void volume, real gas in salt/Reactor, BaCl2//NH3, no walls, with algebraic loops, real gas in void volume, real gas in salt/Reactor (no walls)/Reactor's temperature and pressure/Reactor's energy balance/Void volume pressure equation (real model) ==
  note: The ideal gas model is presented here
      | just for the sake of comparison,
      | but it is not used outside this block.
  In2 : Inport
  In1 : Inport  Port=2
  Gain1 : Gain  Gain=1/V_void
  Ideal gas equation of state : thermochemical/Thermodynamic fluid properties/Ideal gas equation of state  sel=P(T,rho)  R=8.3145  Pa_to_bar=1e-5  bar_to_Pa=1e5
      settings: SourceProductName=@ Thermochemical
  Mux1 : Mux  Inputs=2
  P(T,rho) : thermochemical/Thermodynamic fluid properties/Thermodynamic  property (non-saturated)  sel=P(T,rho)  fluid=fluid  reciprocVar=-1  lookup2D_BreakPoint1=fluid.no_sat.T_rho_indep.var_indep.T  lookup2D_BreakPoint2=fluid.no_sat.T_rho_indep.var_indep.rho_molar  lookup2D_Data=fluid.no_sat.T_rho_indep.var_dep.P
      settings: SourceProductName=@ Thermochemical
  Terminator : Terminator
  Out1 : Outport
  wires:
  Mux1/1 -> Terminator/1  "Comparison"
  Ideal gas equation of state/1 -> Mux1/2  "P_reactor ideal (bar)"
  P(T,rho)/1 -> Mux1/1, Out1/1  "P_reactor (bar)"
  Gain1/1 -> Ideal gas equation of state/2, P(T,rho)/2  "rho_molar (mol/m3)"
  In2/1 -> Ideal gas equation of state/1, P(T,rho)/1  "T (K)"
  In1/1 -> Gain1/1  "N (mol)"

== system thermochemical/Reactors/Reactor, BaCl2//NH3, state-space form, [Tr, Ng, X] as state variables, no algebraic loops, ideal gas in void volume, ideal gas in salt/Reactor, BaCl2//NH3, no walls, state-space form, [Tr, Ng, X] as state variables, no algebraic loops, ideal gas in void volume/Reactor, no walls, state space form/Reactor state-space functions/f1/f3/Reaction kinetic, differential equation ==
  note: Synthesis
  note: Desorption
  In1 : Inport
  In2 : Inport  Port=2
  In3 : Inport  Port=3
  3 : Constant
  Clausius-Clapeyron : thermochemical/Thermodynamic fluid properties/Clausius-Clapeyron  sel_1=P(T)  sel_2=BaCl2/NH3
      settings: SourceProductName=@ Thermochemical
  Divide1 : Product  Inputs=/*
  Gain15 : Gain  Gain=K_cin
  Product6 : Product
  Relay : Relay  OnSwitchValue=P_dead_zone  OffSwitchValue=-P_dead_zone  OffOutputValue=-1
  Sum16 : Sum  Inputs=+-
  Sum17 : Sum  Inputs=+-|
  Switch : Switch  Criteria=u2 > Threshold
  Out2 : Outport
  wires:
  In3/1 -> Switch/3, Sum17/2  "X (0..1)"
  Relay/1 -> Switch/2
  In1/1 -> Clausius-Clapeyron/1  "T(K)"
  Sum16/1 -> Divide1/2, Relay/1  "dP"
  Clausius-Clapeyron/1 -> Sum16/2  "P_equilb (bar)"
  Gain15/1 -> Product6/1
  3/1 -> Sum17/1
  Product6/1 -> Out2/1  "dX/dt"
  In2/1 -> Divide1/1, Sum16/1  "P (bar)"
  Switch/1 -> Product6/2
  Divide1/1 -> Gain15/1
  Sum17/1 -> Switch/1  "1 - X"

== system thermochemical/Reactors/Reactor, BaCl2//NH3, state-space form, [Tr, Ng, X] as state variables, no algebraic loops, ideal gas in void volume, ideal gas in salt/Reactor, BaCl2//NH3, no walls, state-space form, [Tr, Ng, X] as state variables, no algebraic loops, ideal gas in void volume/Reactor, no walls, state space form/Reactor state-space functions/f3/f3/Reaction kinetic, differential equation ==
  note: Synthesis
  note: Desorption
  In1 : Inport
  In2 : Inport  Port=2
  In3 : Inport  Port=3
  3 : Constant
  Clausius-Clapeyron : thermochemical/Thermodynamic fluid properties/Clausius-Clapeyron  sel_1=P(T)  sel_2=BaCl2/NH3
      settings: SourceProductName=@ Thermochemical
  Divide1 : Product  Inputs=/*
  Gain15 : Gain  Gain=K_cin
  Product6 : Product
  Relay : Relay  OnSwitchValue=P_dead_zone  OffSwitchValue=-P_dead_zone  OffOutputValue=-1
  Sum16 : Sum  Inputs=+-
  Sum17 : Sum  Inputs=+-|
  Switch : Switch  Criteria=u2 > Threshold
  Out2 : Outport
  wires:
  In3/1 -> Switch/3, Sum17/2  "X (0..1)"
  Relay/1 -> Switch/2
  In1/1 -> Clausius-Clapeyron/1  "T(K)"
  Sum16/1 -> Divide1/2, Relay/1  "dP"
  Clausius-Clapeyron/1 -> Sum16/2  "P_equilb (bar)"
  Gain15/1 -> Product6/1
  3/1 -> Sum17/1
  Product6/1 -> Out2/1  "dX/dt"
  In2/1 -> Divide1/1, Sum16/1  "P (bar)"
  Switch/1 -> Product6/2
  Divide1/1 -> Gain15/1
  Sum17/1 -> Switch/1  "1 - X"
